simulink subsystem "rss_ElecSpdCtlSens"  (R2023a)
settings: Solver=VariableStepAuto  StartTime=0.0  StopTime=10.0  RelTol=1e-3
undefined symbols (not defined in the file): bit, Cdbl_nElecAgSpdMaxVal, Cdbl_trqTqMaxVal, ENM_MOTO_STATUS, Gs16_trqInitCondTq_C
libraries: simulink x2, lib_configurable_parameter x2, lib_discrete_time_PI_controller x1, lib_discrete_time_PI_controller32bit x1
settings Model: DefaultTestHarness=rss_ElectricSpeedController_SensorBased_thu  Creator=RAN2OFO  LastModifiedBy=xiaoqiang.yuan
settings OptimizationCC: ReuseModelBlockBuffer=off

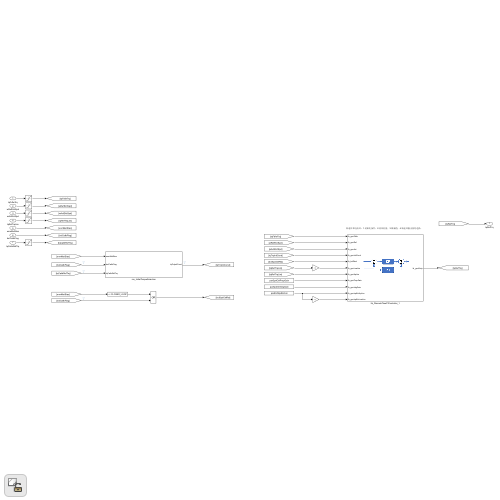
[thumbnail: Simulink's stored preview of the top-level diagram]
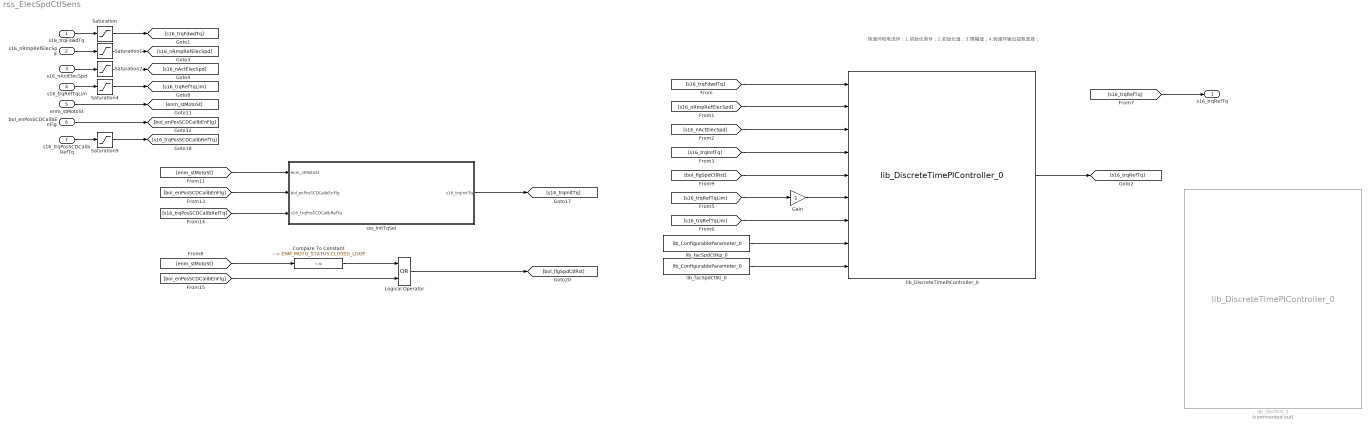
== system rss_ElecSpdCtlSens ==
  note: 转速环和电流环：1.初始化条件；2.初始化值；3.限幅值；4.转速环输出扭矩选择；
  s16_trqFdwdTq : Inport  OutDataTypeStr=dt_Standardize_s16p15b0
  s16_nRmpRefElecSpd : Inport  Port=2  OutDataTypeStr=dt_Standardize_s16p15b0
  s16_nActElecSpd : Inport  Port=3  OutDataTypeStr=dt_Standardize_s16p15b0
  s16_trqRefTqLim : Inport  Port=4  OutDataTypeStr=dt_Standardize_s16p15b0
  enm_stMotoSt : Inport  Port=5  OutDataTypeStr=Enum: ENM_MOTO_STATUS
  bol_enPosSCDCalibEnFlg : Inport  Port=6  OutDataTypeStr=boolean
  s16_trqPosSCDCalibRefTq : Inport  Port=7  OutDataTypeStr=dt_Standardize_s16p15b0
  Compare To Constant : simulink/Logic and Bit Operations/Compare To Constant  relop=~=  const=ENM_MOTO_STATUS.CLOSED_LOOP  OutDataTypeStr=boolean
  Gain : Gain  Gain=-1  RndMeth=Simplest  OutDataTypeStr=Inherit: Same as input
  Logical Operator : Logic  Operator=OR  AllPortsSameDT=off  OutDataTypeStr=boolean
  Saturation : Saturate  UpperLimit=Cdbl_trqTqMaxVal  LowerLimit=-Cdbl_trqTqMaxVal
  Saturation1 : Saturate  UpperLimit=Cdbl_nElecAgSpdMaxVal  LowerLimit=-Cdbl_nElecAgSpdMaxVal
  Saturation2 : Saturate  UpperLimit=Cdbl_nElecAgSpdMaxVal  LowerLimit=-Cdbl_nElecAgSpdMaxVal
  Saturation4 : Saturate  UpperLimit=Cdbl_trqTqMaxVal  LowerLimit=-Cdbl_trqTqMaxVal
  Saturation9 : Saturate  UpperLimit=Cdbl_trqTqMaxVal  LowerLimit=-Cdbl_trqTqMaxVal
  lib_DisTiCtl_1 : lib_discrete_time_PI_controller/lib_DiscreteTimePIController_0  Commented=on  lb_parSampTime=Cu16_tiSlwTaskSmpTi  lb_parMaxSampTime=0.1  lb_parMaxPropGain=Cdbl_facSpdCtlKpMaxVal  lb_parMaxIntgGain=Cdbl_facSpdCtlKiMaxVal  lb_parRefInpMaxVal=Cdbl_nElecAgSpdMaxVal  lb_parRefInpMinVal=-Cdbl_nElecAgSpdMaxVal  lb_parMaxErrVal=2*Cdbl_nElecAgSpdMaxVal  lb_parMinErrVal=-2*Cdbl_nElecAgSpdMaxVal  lb_parMaxOutpVal=Cdbl_trqTqMaxVal  lb_parMinOutpVal=-Cdbl_trqTqMaxVal  lb_parAccmDataTypeMode=32-bit  lb_parOutpDataType=dt_Standardize_s16p15b0  lb_parSatMode=anti-windup with back-calculation
  lib_DiscreteTimePIController_0 : lib_discrete_time_PI_controller32bit/lib_DiscreteTimePIController_0  lb_parSampTime=Cdbl_tiSlwTaskSmpTi  lb_parMaxSampTime=0.1  lb_parMaxPropGain=Cdbl_facSpdCtlKpMaxVal  lb_parMaxIntgGain=Cdbl_facSpdCtlKiMaxVal  lb_parRefInpMaxVal=Cdbl_nElecAgSpdMaxVal  lb_parRefInpMinVal=-Cdbl_nElecAgSpdMaxVal  lb_parMaxErrVal=2*Cdbl_nElecAgSpdMaxVal  lb_parMinErrVal=-2*Cdbl_nElecAgSpdMaxVal  lb_parMaxOutpVal=Cdbl_trqTqMaxVal  lb_parMinOutpVal=-Cdbl_trqTqMaxVal  lb_parAccmDataTypeMode=32-bit  lb_parOutpDataType=dt_Standardize_s16p15b0  lb_parSatMode=anti-windup with back-calculation
  lib_facSpdCtlKi_0 : lib_configurable_parameter/lib_ConfigurableParameter_0  lb_parCnfgPar=Gu16_facSpdCtlKi_C  lb_parDataType=Inherit: Inherit from 'Constant value'  lb_parUpLim=Cdbl_facSpdCtlKiMaxVal  lb_parLowLim=0
  lib_facSpdCtlKp_0 : lib_configurable_parameter/lib_ConfigurableParameter_0  lb_parCnfgPar=Gu16_facSpdCtlKp_C  lb_parDataType=Inherit: Inherit from 'Constant value'  lb_parUpLim=Cdbl_facSpdCtlKpMaxVal  lb_parLowLim=0
  sss_InitTqSel : Subsystem  VariantControl=cstSensCtrlLbl
  s16_trqRefTq : Outport  OutDataTypeStr=dt_Standardize_s16p15b0
  wires:
  [s16_trqRefTqLim] -> Gain/1
  s16_trqFdwdTq/1 -> Saturation/1
  [s16_trqInitTq] -> lib_DiscreteTimePIController_0/4
  s16_trqRefTqLim/1 -> Saturation4/1
  [s16_nRmpRefElecSpd] -> lib_DiscreteTimePIController_0/2
  [s16_nActElecSpd] -> lib_DiscreteTimePIController_0/3
  [s16_trqFdwdTq] -> lib_DiscreteTimePIController_0/1
  Saturation4/1 -> [s16_trqRefTqLim]
  lib_DiscreteTimePIController_0/1 -> [s16_trqRefTq]
  Saturation1/1 -> [s16_nRmpRefElecSpd]
  [bol_flgSpdCtlRst] -> lib_DiscreteTimePIController_0/5
  s16_nRmpRefElecSpd/1 -> Saturation1/1
  [s16_trqRefTqLim] -> lib_DiscreteTimePIController_0/7
  s16_nActElecSpd/1 -> Saturation2/1
  Gain/1 -> lib_DiscreteTimePIController_0/6
  [enm_stMotoSt] -> Compare To Constant/1
  Saturation2/1 -> [s16_nActElecSpd]
  Saturation/1 -> [s16_trqFdwdTq]
  sss_InitTqSel/1(s16_trqInitTq) -> [s16_trqInitTq]
  Compare To Constant/1 -> Logical Operator/1
  Logical Operator/1 -> [bol_flgSpdCtlRst]
  [bol_enPosSCDCalibEnFlg] -> Logical Operator/2
  s16_trqPosSCDCalibRefTq/1 -> Saturation9/1
  enm_stMotoSt/1 -> [enm_stMotoSt]
  Saturation9/1 -> [s16_trqPosSCDCalibRefTq]
  bol_enPosSCDCalibEnFlg/1 -> [bol_enPosSCDCalibEnFlg]
  [enm_stMotoSt] -> sss_InitTqSel/1(enm_stMotoSt)
  [bol_enPosSCDCalibEnFlg] -> sss_InitTqSel/2(bol_enPosSCDCalibEnFlg)
  [s16_trqPosSCDCalibRefTq] -> sss_InitTqSel/3(s16_trqPosSCDCalibRefTq)
  [s16_trqRefTq] -> s16_trqRefTq/1
  lib_facSpdCtlKp_0/1 -> lib_DiscreteTimePIController_0/8
  lib_facSpdCtlKi_0/1 -> lib_DiscreteTimePIController_0/9

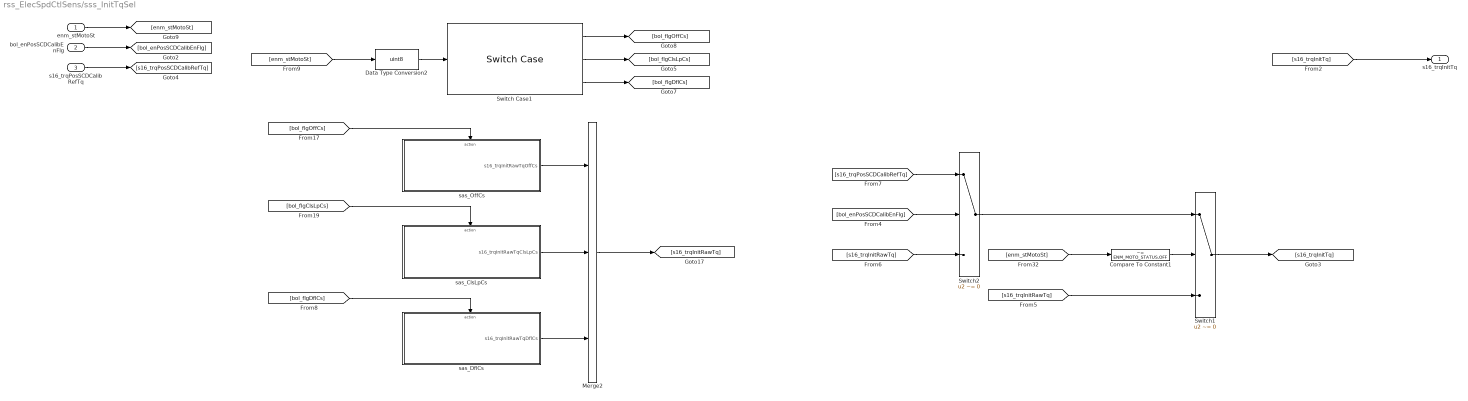
== system rss_ElecSpdCtlSens/sss_InitTqSel ==
  enm_stMotoSt : Inport
  bol_enPosSCDCalibEnFlg : Inport  Port=2
  s16_trqPosSCDCalibRefTq : Inport  Port=3
  Compare To Constant1 : simulink/Logic and Bit Operations/Compare To Constant  relop=~=  const=ENM_MOTO_STATUS.OFF  OutDataTypeStr=boolean
  Data Type Conversion2 : DataTypeConversion  OutDataTypeStr=uint8  SaturateOnIntegerOverflow=off  RndMeth=Floor
  Merge2 : Merge  Inputs=3
  Switch Case1 : SwitchCase  CaseConditions={0,2}
  Switch1 : Switch  Criteria=u2 ~= 0  SaturateOnIntegerOverflow=off  InputSameDT=off
  Switch2 : Switch  Criteria=u2 ~= 0  SaturateOnIntegerOverflow=off  InputSameDT=off
  sas_ClsLpCs : Subsystem  TreatAsAtomicUnit=on
  sas_DflCs : Subsystem  TreatAsAtomicUnit=on
  sas_OffCs : Subsystem  TreatAsAtomicUnit=on
  s16_trqInitTq : Outport
  wires:
  Switch Case1/1 -> [bol_flgOffCs]
  Merge2/1 -> [s16_trqInitRawTq]
  [bol_flgClsLpCs] -> sas_ClsLpCs/Action
  [bol_flgDflCs] -> sas_DflCs/Action
  sas_OffCs/1(s16_trqInitRawTqOffCs) -> Merge2/1
  Switch Case1/2 -> [bol_flgClsLpCs]
  sas_ClsLpCs/1(s16_trqInitRawTqClsLpCs) -> Merge2/2
  [bol_flgOffCs] -> sas_OffCs/Action
  Data Type Conversion2/1 -> Switch Case1/1
  [enm_stMotoSt] -> Data Type Conversion2/1
  Switch Case1/3 -> [bol_flgDflCs]
  sas_DflCs/1(s16_trqInitRawTqDflCs) -> Merge2/3
  s16_trqPosSCDCalibRefTq/1 -> [s16_trqPosSCDCalibRefTq]
  [s16_trqPosSCDCalibRefTq] -> Switch2/1
  [s16_trqInitRawTq] -> Switch2/3
  Switch2/1 -> Switch1/1
  [s16_trqInitRawTq] -> Switch1/3
  [bol_enPosSCDCalibEnFlg] -> Switch2/2
  Switch1/1 -> [s16_trqInitTq]
  Compare To Constant1/1 -> Switch1/2
  [enm_stMotoSt] -> Compare To Constant1/1
  bol_enPosSCDCalibEnFlg/1 -> [bol_enPosSCDCalibEnFlg]
  enm_stMotoSt/1 -> [enm_stMotoSt]
  [s16_trqInitTq] -> s16_trqInitTq/1

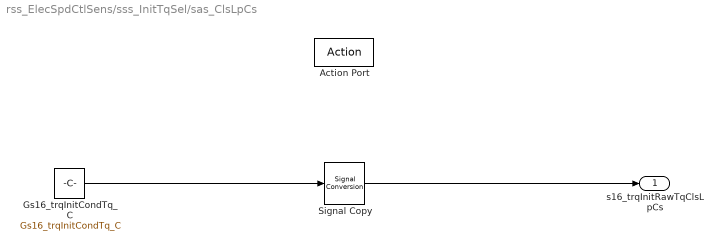
== system rss_ElecSpdCtlSens/sss_InitTqSel/sas_ClsLpCs ==
  Action Port : ActionPort
  Gs16_trqInitCondTq_C : Constant  Value=Gs16_trqInitCondTq_C
  Signal Copy : SignalConversion  OverrideOpt=off
  s16_trqInitRawTqClsLpCs : Outport
  wires:
  Signal Copy/1 -> s16_trqInitRawTqClsLpCs/1
  Gs16_trqInitCondTq_C/1 -> Signal Copy/1

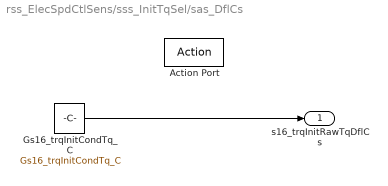
== system rss_ElecSpdCtlSens/sss_InitTqSel/sas_DflCs ==
  Action Port : ActionPort
  Gs16_trqInitCondTq_C : Constant  Value=Gs16_trqInitCondTq_C
  s16_trqInitRawTqDflCs : Outport
  wires:
  Gs16_trqInitCondTq_C/1 -> s16_trqInitRawTqDflCs/1

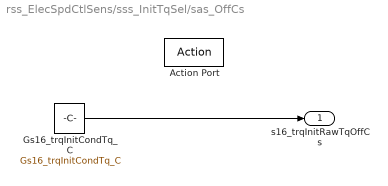
== system rss_ElecSpdCtlSens/sss_InitTqSel/sas_OffCs ==
  Action Port : ActionPort
  Gs16_trqInitCondTq_C : Constant  Value=Gs16_trqInitCondTq_C
  s16_trqInitRawTqOffCs : Outport
  wires:
  Gs16_trqInitCondTq_C/1 -> s16_trqInitRawTqOffCs/1
